simulink model "untitled2"  (R2018b)
settings: Solver=FixedStepAuto  StartTime=0.0  StopTime=inf  RelTol=1e-3  EnableMultiTasking=on
libraries: mbedblockslib x3
settings Model: Creator=hpong  LastModifiedBy=hpong
settings OptimizationCC: EnhancedBackFolding=on  PassReuseOutputArgsAs=Individual arguments  MaxStackSize=64  OptimizeBlockOrder=speed  DifferentSizesBufferReuse=on  OptimizationCustomize=off
settings DebuggingCC: ParameterTunabilityLossMsg=error
settings HardwareCC: ProdBitPerPointer=32  ProdBitPerSizeT=32  ProdBitPerPtrDiffT=32  ProdLargestAtomicInteger=Long  ProdLargestAtomicFloat=Double  ProdWordSize=32  ProdHWDeviceType=ARM Compatible->ARM Cortex
settings SFSimCC: MATLABDynamicMemAlloc=off
settings RTWCC: SystemTargetFile=ert.tlc  HardwareBoard=STM32F769I-Discovery  TemplateMakefile=ert_default_tmf  GenerateReport=on  Toolchain=GNU Tools for ARM Embedded Processors  IncludeHyperlinkInReport=on  LaunchReport=on  GenerateTraceInfo=on  GenerateTraceReport=on  GenerateTraceReportSl=on  GenerateTraceReportSf=on  GenerateTraceReportEml=on
settings CodeAppCC: ForceParamTrailComments=on  IgnoreCustomStorageClasses=off  OperatorAnnotations=on  SimulinkDataObjDesc=on  SFDataObjDesc=on  InsertBlockDesc=on
settings ERTTargetCC: CodeReplacementLibrary=ARM Cortex-M (CMSIS)

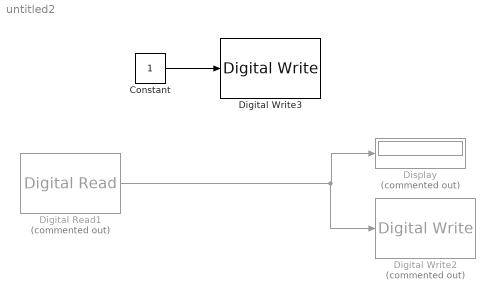
== system untitled2 ==
  Constant : Constant  SampleTime=1
  Digital Read1 : mbedblockslib/Digital Read  Commented=on  Pin=PA_0  Direction=input  SampleTime=0.1
      settings: SourceProductName=Simulink Coder Support Package for BBC microbit Board  SourceProductBaseCode=MICROBIT
  Digital Write2 : mbedblockslib/Digital Write  Commented=on  Pin=PA_13  Direction=output
      settings: SourceProductName=Simulink Coder Support Package for BBC microbit Board  SourceProductBaseCode=MICROBIT
  Digital Write3 : mbedblockslib/Digital Write  Pin=PJ_13  Direction=output
      settings: SourceProductName=Simulink Coder Support Package for BBC microbit Board  SourceProductBaseCode=MICROBIT
  Display : Display  Commented=on
  wires:
  Digital Read1/1 -> Digital Write2/1, Display/1
  Constant/1 -> Digital Write3/1
